simulink model "test"  (R2023b)
settings: Solver=FixedStepAuto  StartTime=0.0  StopTime=inf  FixedStep=0.01  RelTol=1e-3
settings Model: Creator=branko  LastModifiedBy=branko

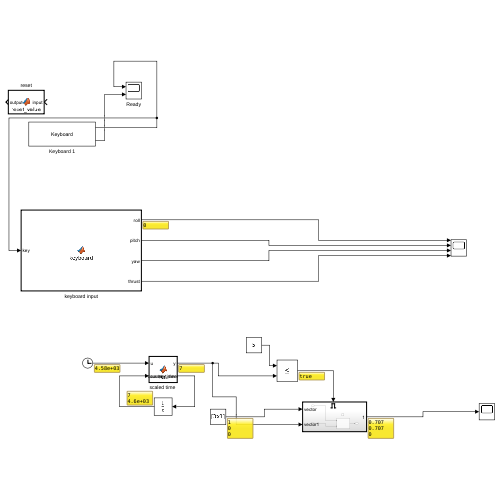
[thumbnail: Simulink's stored preview of the top-level diagram]
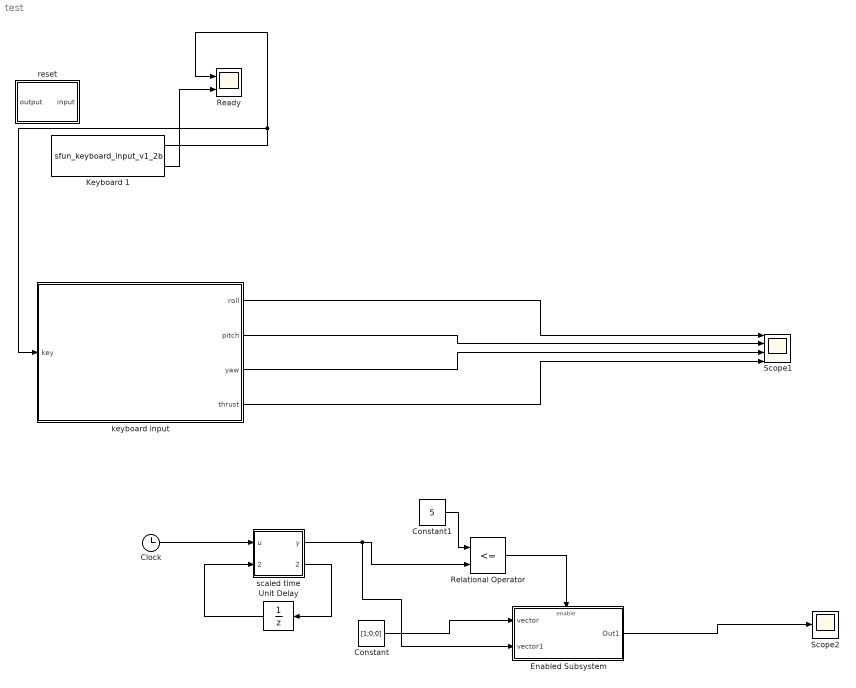
== system test ==
  Clock : Clock
  Constant : Constant  Value=[1;0;0]
  Constant1 : Constant  Value=5
  Enabled Subsystem : Subsystem  TreatAsAtomicUnit=on
  Keyboard 1 : M-S-Function  FunctionName=sfun_keyboard_input_v1_2b  mask(Keyboard Input){}
      mask help: Keyboard Input
      mask Display: fprintf('Keyboard');
  Ready : Scope  NumInputPorts=2
  Relational Operator : RelationalOperator  Operator=<=  OutDataTypeStr=boolean  RndMeth=Simplest  InputSameDT=off
  Scope1 : Scope  NumInputPorts=4
  Scope2 : Scope
  Unit Delay : UnitDelay  InitialCondition=[0 25]  SampleTime=0.01  HasFrameUpgradeWarning=on
  keyboard input : MATLAB Function  TreatAsAtomicUnit=on
  reset : MATLAB Function  TreatAsAtomicUnit=on
  "scaled time " : MATLAB Function  TreatAsAtomicUnit=on
  wires:
  keyboard input/2(pitch) -> Scope1/2
  keyboard input/3(yaw) -> Scope1/3
  keyboard input/4(thrust) -> Scope1/4
  Keyboard 1/2 -> Ready/2
  keyboard input/1(roll) -> Scope1/1
  Keyboard 1/1 -> Ready/1, keyboard input/1(key)
  Constant1/1 -> Relational Operator/1
  Relational Operator/1 -> Enabled Subsystem/Enable
  Enabled Subsystem/1(Out1) -> Scope2/1
  Constant/1 -> Enabled Subsystem/1(vector)
  "scaled time "/1(y) -> Enabled Subsystem/2(vector1), Relational Operator/2
  Clock/1 -> "scaled time "/1(u)
  "scaled time "/2(counter_timer) -> Unit Delay/1
  Unit Delay/1 -> "scaled time "/2("counter_timer ")

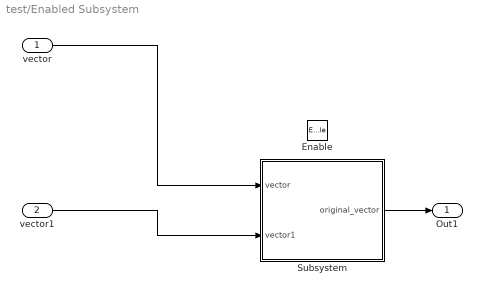
== system test/Enabled Subsystem ==
  vector : Inport
  vector1 : Inport  Port=2
  Enable : EnablePort
  Subsystem : Subsystem
  Out1 : Outport
  wires:
  vector/1 -> Subsystem/1(vector)
  Subsystem/1(original_vector) -> Out1/1
  vector1/1 -> Subsystem/2(vector1)

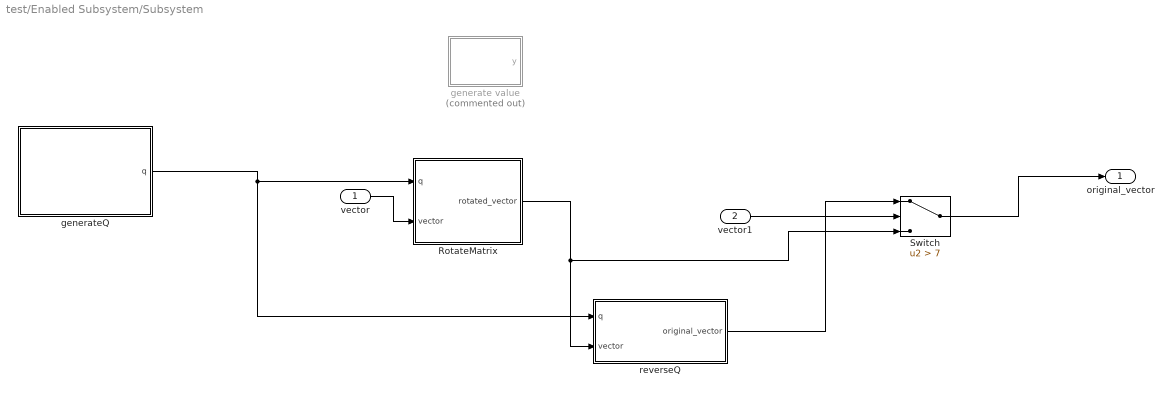
== system test/Enabled Subsystem/Subsystem ==
  vector : Inport
  vector1 : Inport  Port=2
  " generateQ" : MATLAB Function  TreatAsAtomicUnit=on
  RotateMatrix : MATLAB Function  TreatAsAtomicUnit=on
  Switch : Switch  Criteria=u2 > Threshold  Threshold=7  SaturateOnIntegerOverflow=off  InputSameDT=off
  generate value : MATLAB Function  Commented=on  TreatAsAtomicUnit=on
  reverseQ : MATLAB Function  TreatAsAtomicUnit=on
  original_vector : Outport
  wires:
  vector/1 -> RotateMatrix/2(vector)
  " generateQ"/1(q) -> reverseQ/1(q), RotateMatrix/1(q)
  RotateMatrix/1(rotated_vector) -> reverseQ/2(vector), Switch/3
  Switch/1 -> original_vector/1
  vector1/1 -> Switch/2
  reverseQ/1(original_vector) -> Switch/1

== matlab function test/Enabled Subsystem/Subsystem/RotateMatrix ==
  data: q input; rotated_vector output; vector input
function rotated_vector = applyQuaternionRotation(q, vector)
    % quaternion components
    w = q(1);
    x = q(2);
    y = q(3);
    z = q(4);
    % Quaternion rotation matrix
    R = [1 - 2*y^2 - 2*z^2, 2*x*y - 2*z*w, 2*x*z + 2*y*w;
         2*x*y + 2*z*w, 1 - 2*x^2 - 2*z^2, 2*y*z - 2*x*w;
         2*x*z - 2*y*w, 2*y*z + 2*x*w, 1 - 2*x^2 - 2*y^2];
    % rotate
    rotated_vector = R * vector;
end

== matlab function test/Enabled Subsystem/Subsystem/ generateQ ==
  data: q output
function q = generateQuaternion()
    %angle in radians (45 degrees) or beta
    angle_radians = deg2rad(45);
    % Fixed axis 
    axis = [0; 0; 1];
    % Calculate the quaternion
    q = [cos(angle_radians / 2); sin(angle_radians / 2) * axis];
end

== matlab function test/Enabled Subsystem/Subsystem/reverseQ ==
  data: q input; original_vector output; vector input
function original_vector = revertQuaternionRotation(q, vector)
    % Extract quaternion components
    w = q(1);
    x = -q(2);
    y = -q(3);
    z = -q(4);
    % Inverse quaternion (conjugate for unit quaternion)
    % Apply inverse rotation
     % Quaternion rotation matrix again but with the inverse quartonion
     % this time
    R = [1 - 2*y^2 - 2*z^2, 2*x*y - 2*z*w, 2*x*z + 2*y*w;
         2*x*y + 2*z*w, 1 - 2*x^2 - 2*z^2, 2*y*z - 2*x*w;
         2*x*z - 2*y*w, 2*y*z + 2*x*w, 1 - 2*x^2 - 2*y^2];
    % Apply rotation on the inverse
    original_vector = R * vector;
end

== matlab function test/Enabled Subsystem/Subsystem/generate value ==
  data: y output
function y = random_counter()
    persistent counter;
    
    % Initialize counter if not already initialized
    if isempty(counter)
        counter = 0;
    end
    
    % Increment counter
    counter = counter + 1;
    display(counter)
    % Check if counter has reached a random interval between 0 and 20
    if counter >= 2
        
        % Reset counter to 0
        counter = 0;
    end
    
    y = counter;
end

== matlab function test/keyboard input ==
  data: roll output; pitch output; yaw output; thrust output; key input
 function [roll, pitch, yaw, thrust] = keyboard(key)
    pitch_increment = 0.1;
    roll_increment = 0.1;
    yaw_increment = 0.1;
    thrust_increment = 0.1;
    
    % Initialize

    roll = 0;
    pitch = 0;
    yaw = 0;
    thrust = 0;

   
    persistent prev_roll prev_pitch prev_yaw prev_thrust counter;
    
    
    if isempty(prev_roll), prev_roll = 0; end
    if isempty(prev_pitch), prev_pitch = 0; end
    if isempty(prev_yaw), prev_yaw = 0; end
    if isempty(prev_thrust), prev_thrust = 0; end
    if isempty(counter), counter = 0; end
    
   
    switch key
        case 119  % 'w'
            pitch = prev_pitch + pitch_increment; % Increase pitch
            counter = counter + 1;
        case 115  % 's'
            pitch = prev_pitch - pitch_increment; % Decrease pitch
              counter = counter +1;
        case 97   % 'a'
            roll = prev_roll - roll_increment; % Decrease roll
              counter = counter +1;
        case 100  % 'd'
            roll = prev_roll + roll_increment; % Increase roll
              counter = counter +1;
        case 32   % Space key
            thrust = prev_thrust + thrust_increment; % Increase thrust
              counter = counter +1;
        case 113  % 'q'
            yaw = prev_yaw - yaw_increment; % Decrease yaw
              counter = counter + 1;
        case 101  % 'e'
            yaw = prev_yaw + yaw_increment; % Increase yaw
            counter = counter +1;
        
        otherwise
            
      
            roll = prev_roll;
            pitch = prev_pitch;
            yaw = prev_yaw;
            thrust = prev_thrust;
        
          
       
   
            return;
    end
    
    % Bound roll, pitch, yaw, and thrust range
    roll = max(min(roll, 1), -1);
    pitch = max(min(pitch, 1), -1);
    yaw = max(min(yaw, 1), -1);
    thrust = max(min(thrust, 1), 0); % Thrust 
    
    % next iteration
    prev_roll = roll;
    prev_pitch = pitch;
    prev_yaw = yaw;
    prev_thrust = thrust;
end

== matlab function test/reset ==
  data: input input; output output
function output = reset_value(input)
    % Used value
    persistent used;
    if isempty(used)
       
        used = false;
    end
    
    
    if ~used
        output = input;
       
        used = true;
    else
        output = 0;
    end
end

== matlab function test/scaled time  ==
  data: u input; counter_timer input; y output; counter_timer output
function [y,counter_timer] = fcn(u,counter_timer)
 
if u == counter_timer(2)
   counter_timer(1) = counter_timer(1) +1; 
   counter_timer(2) = counter_timer(2) + 25;
      
end
if counter_timer(1) == 11
  counter_timer(1) = 0;
end

y = counter_timer(1);
